simulink model "model1"  (R2023a)
settings: Solver=ode45  StartTime=0.0  StopTime=4  FixedStep=dt  MaxStep=0.001  RelTol=1e-3
values from neighbouring files (symbols this model uses):
  IC = [track_len/2, pi, 0, 0]'    [ALLINONE.m]    (also in main1_finHorLQR_OperatingPoint.m = [track_len/2;the0deg*pi/180;0;0]; main2_finHorLQR_program_Trajectory.m = [track_len/2;the0deg*pi/180;0;0])
settings Model: Creator=Adam  LastModifiedBy=domrazek
settings SolverCC: AlgebraicLoopSolver=TrustRegion
settings DataIOCC: ExternalInput=ind1  LoadExternalInput=on  SignalLogging=off  DSMLogging=off  OutputSaveName=out  ReturnWorkspaceOutputsName=sout
settings OptimizationCC: SimCompilerOptimization=on  AccelVerboseBuild=on
settings DebuggingCC: AlgebraicLoopMsg=none  UnconnectedInputMsg=warning  UnconnectedOutputMsg=warning  UnconnectedLineMsg=warning
settings ModelReferenceCC: EnableRefExpFcnMdlSchedulingChecks=on
settings RTWCC: DLArmComputeVersion=19.05

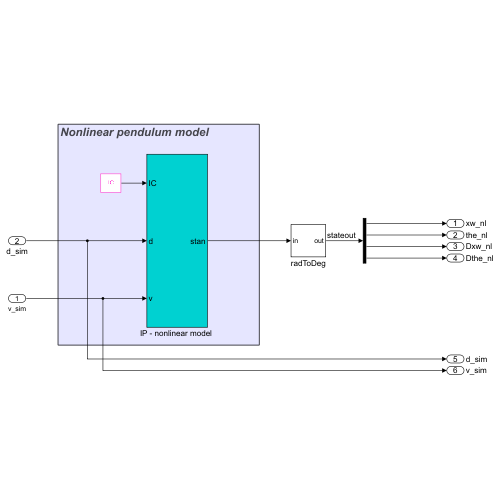
[thumbnail: Simulink's stored preview of the top-level diagram]
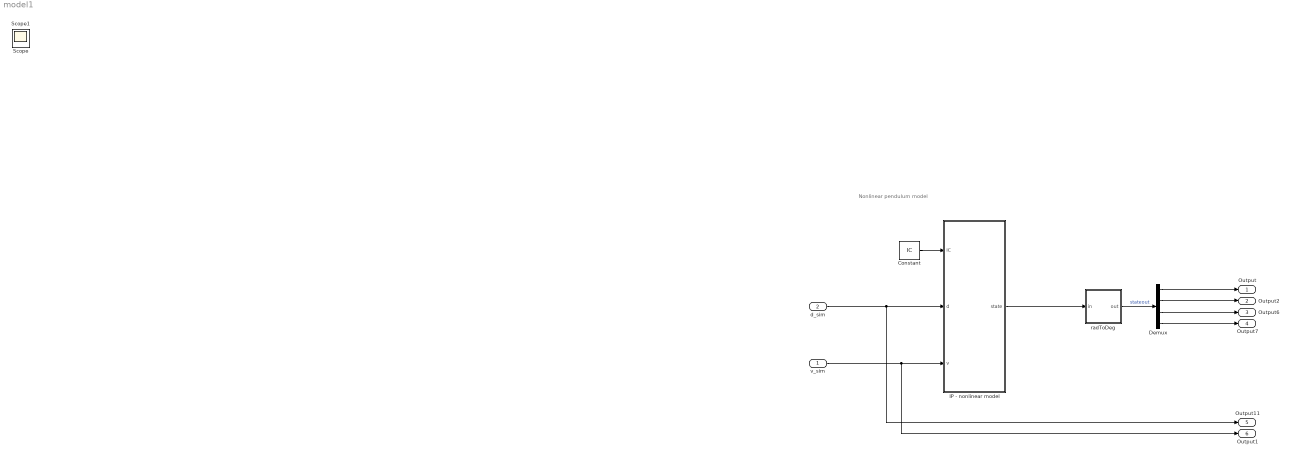
== system model1 ==
  note: Nonlinear pendulum model
  v_sim : Inport
  d_sim : Inport  Port=2
  Constant : Constant  Value=IC  VectorParams1D=off
  Demux : Demux
  "IP - nonlinear model " : Subsystem  Description=Nonlinear model of inverted pendulum
      mask Display:
      | port_label('output', 1, 'stan');
      | port_label('input', 1, 'IC');
      | port_label('input', 2, 'd');
      | port_label('input', 3, 'v');
  radToDeg : Subsystem
  Output : Outport  SignalName=xw_nl
  Output2 : Outport  Port=2  SignalName=the_nl
  Output6 : Outport  Port=3  SignalName=Dxw_nl
  Output7 : Outport  Port=4  SignalName=Dthe_nl
  Output11 : Outport  Port=5  SignalName=d_sim
  Output1 : Outport  Port=6  SignalName=v_sim
  Scope : Scope
  Scope1 : Scope
  wires:
  "IP - nonlinear model "/1(state) -> radToDeg/1(in)
  Constant/1 -> "IP - nonlinear model "/1(IC)
  d_sim/1 -> "IP - nonlinear model "/2(d), Output11/1
  radToDeg/1(out) -> Demux/1  "stateout"
  Demux/1 -> Output/1
  Demux/2 -> Output2/1
  Demux/3 -> Output6/1
  Demux/4 -> Output7/1
  v_sim/1 -> Output1/1, "IP - nonlinear model "/3(v)

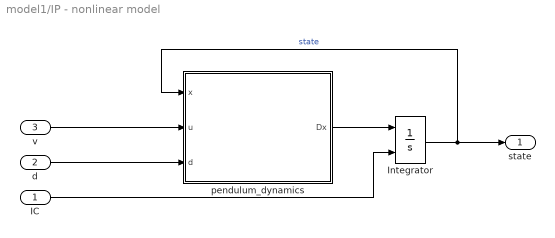
== system model1/IP - nonlinear model  ==
  IC : Inport
  d : Inport  Port=2
  v : Inport  Port=3
  Integrator : Integrator  InitialConditionSource=external
  pendulum_dynamics : MATLAB Function  TreatAsAtomicUnit=on
  state : Outport
  wires:
  Integrator/1 -> state/1, pendulum_dynamics/1(x)  "state"
  v/1 -> pendulum_dynamics/2(u)
  pendulum_dynamics/1(Dx) -> Integrator/1
  IC/1 -> Integrator/2
  d/1 -> pendulum_dynamics/3(d)

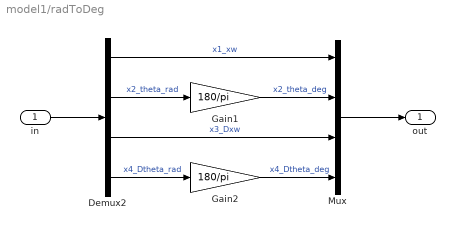
== system model1/radToDeg ==
  in : Inport
  Demux2 : Demux
  Gain1 : Gain  Gain=180/pi
  Gain2 : Gain  Gain=180/pi
  Mux : Mux
  out : Outport
  wires:
  Demux2/1 -> Mux/1  "x1_xw"
  Gain1/1 -> Mux/2  "x2_theta_deg"
  Gain2/1 -> Mux/4  "x4_Dtheta_deg"
  Demux2/2 -> Gain1/1  "x2_theta_rad"
  in/1 -> Demux2/1
  Demux2/3 -> Mux/3  "x3_Dxw"
  Demux2/4 -> Gain2/1  "x4_Dtheta_rad"
  Mux/1 -> out/1

== matlab function model1/IP - nonlinear model /pendulum_dynamics ==
  data: x input; u input; d input; Dx output; params_lepkie parameter
function Dx = dynamika_wahadla(x, u, d, params_lepkie)
% x : stan
% u : input - napięcie
%
% params scope: "parameters"
%

% State, function input: x = [x Dx theta Dtheta]'
x1 = x(1);
x2 = x(2); 
x3 = x(3);
x4 = x(4);

params_lepkie = num2cell(params_lepkie);
[M, mc, mp, Lp, Lc, g, b, gamma, mr, Mt, L, Jcm, Jt, alpha, beta] = params_lepkie{:};

% Equations for pendulum dynamics
Ff = b*x3;
Fi = alpha*u - beta*x3;
A = d*cos(x2) - Ff + L*mr*x4^2*sin(x2) + Fi;
B = d*Lc + L*g*mr*sin(x2) - gamma*x4;
DEN = Jt*Mt - (L*mr*cos(x2))^2;

ddt_x1 = x3;
ddt_x2 = x4;
ddt_x3 = (Jt*A - L*mr*cos(x2)*B) / DEN;
ddt_x4 = (Mt*B - L*mr*cos(x2)*A) / DEN;

% output (wektor kolumnowy)
Dx = [ddt_x1 ddt_x2 ddt_x3 ddt_x4]';

end
